simulink model "MATLAB Simulation By Lara"  (R2024a)
settings: Solver=VariableStepAuto  StartTime=0.0  StopTime=20  RelTol=1e-3
undefined symbols (not defined in the file or in its folder): Ion, Lithium
libraries: spsIdealSwitchLib x5, spsSeriesRLCBranchLib x5, instrumentseriallib x2, spsBatteryLib x1, svdutilitieslib x1, spsCurrentMeasurementLib x1, spsDCVoltageSourceLib x1, spsGroundLib x1, spsPVArrayLib x1, spsVoltageMeasurementLib x1, sps_lib x1
settings Model: Creator=LaraW  LastModifiedBy=LaraW

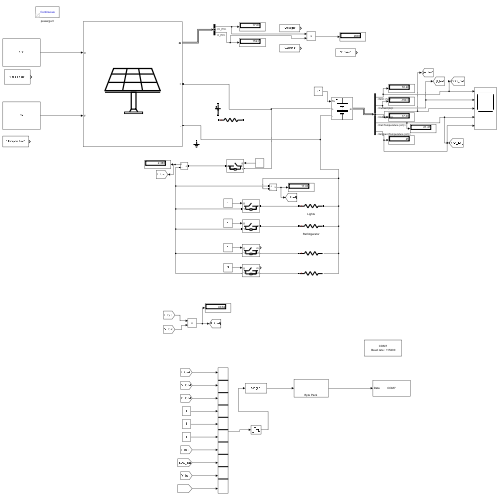
[thumbnail: Simulink's stored preview of the top-level diagram]
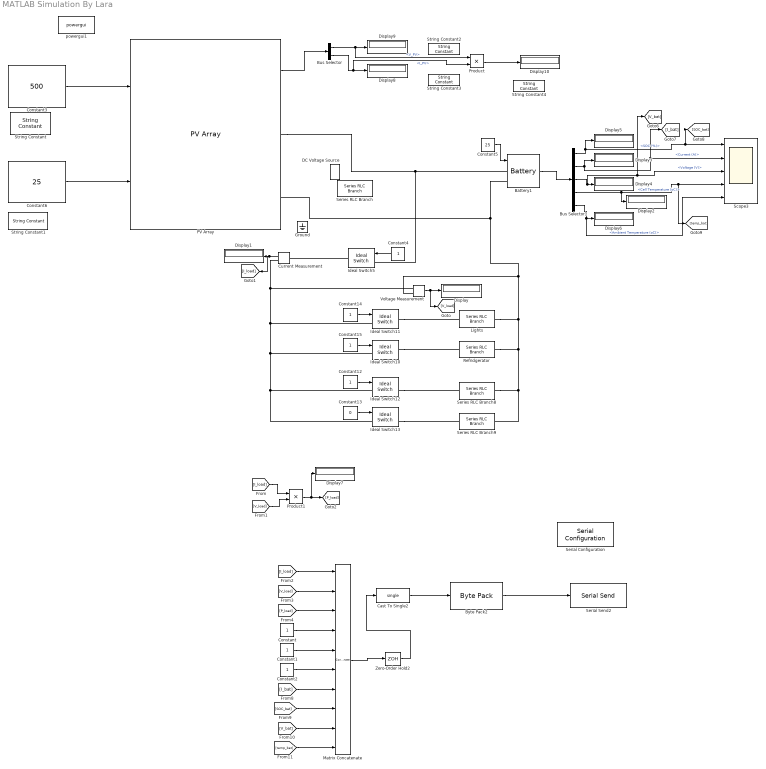
== system MATLAB Simulation By Lara ==
  Battery1 : spsBatteryLib/Battery  BatType=Lithium-Ion  ShowTempParam=on  ThermalPreset="12.8V  40Ah  (LiFeMgPO4)"  ShowAgeParam=off  NomV=12.6  NomQ=40  SOC=70  Batt_Tr=30  PresetModel=off  MaxQ=40  MinV=10.5  FullV=13.8  Dis_rate=20  R=0.015  Normal_OP=30.14  expZone="[13.1          0.5]"  current=[6.5 13 32.5]  Units=Time  Tci=20  NomT=20  T2=0  MaxQ2=36  FullV2=13  Normal_OP2=11.7  expZone2="[12.67            4]"  Rca=0.6411  ti=4880  Dp=0  Neq0=0  Tsim=1e6  Ta1=25  Qeol=5.4*0.9  Reol=0.013333*1.2  Char_age=[2.3478, 3]  Dis_age=[2.3478, 10]  N1=1500  N2=10500  N3=1000  N4=1400  Ta2=45  N5=950
  Bus Selector : BusSelector  OutputSignals=V_PV,I_PV
  Bus Selector1 : BusSelector  OutputSignals=SOC (%),Current (A),Voltage (V),Cell Temperature (oC),Ambient Temperature (oC)
  Byte Pack2 : svdutilitieslib/Byte Pack  maskPackedDataType=uint8  datatypes={'single'}  byteAlign=1  blockPlatform=arduinoert
      settings: LibrarySourceBlock=mcblib/Signal Management/Byte Pack
  Cast To Single2 : DataTypeConversion  OutDataTypeStr=single  SaturateOnIntegerOverflow=off  RndMeth=Floor
  Constant{,1..2,4,12,14..15} (7 alike) : Constant
  Constant13 : Constant  Value=0
  Constant3 : Constant  Value=500
  Constant5 : Constant  Value=25
  Constant6 : Constant  Value=25
  Current Measurement : spsCurrentMeasurementLib/Current Measurement  PhasorSimulation=off  OutputType=Complex  PSBequivalent=0
  DC Voltage Source : spsDCVoltageSourceLib/DC Voltage Source  Amplitude=12  Measurements=None
  Display{,1..10} (11 alike) : Display
  Ground : spsGroundLib/Ground  LConnTagsString=a
  Ideal Switch10 : spsIdealSwitchLib/Ideal Switch  Ron=0.001  Lon=0  IC=0  Rs=1e5  Cs=inf  Measurements=off
  Ideal Switch11 : spsIdealSwitchLib/Ideal Switch  Ron=0.001  Lon=0  IC=0  Rs=1e5  Cs=inf  Measurements=off
  Ideal Switch12 : spsIdealSwitchLib/Ideal Switch  Ron=0.001  Lon=0  IC=0  Rs=1e5  Cs=inf  Measurements=on
  Ideal Switch13 : spsIdealSwitchLib/Ideal Switch  Ron=0.001  Lon=0  IC=0  Rs=1e5  Cs=inf  Measurements=on
  Ideal Switch5 : spsIdealSwitchLib/Ideal Switch  Ron=0.001  Lon=0  IC=0  Rs=1e5  Cs=inf  Measurements=off
  Lights : spsSeriesRLCBranchLib/Series RLC Branch  LConnTagsString=__new0  RConnTagsString=__new0  BranchType=R  Resistance=16  Inductance=1e-3  SetiL0=off  InitialCurrent=0  Capacitance=1e-6  Setx0=off  InitialVoltage=0  Measurements=None
  Matrix Concatenate : Concatenate  NumInputs=10  ConcatenateDimension=2
  PV Array : spsPVArrayLib/PV Array  Npar=50  Nser=1  PlotType=array @ 1000 W/m2 & specified temperatures  S_vec="[ 1000  500  100 ]"  Temp_C_vec="[ 45 25  ]"  ModuleName=User-defined  PlotWhenSelected=off  Pm=110.25  Ncell=20  Voc=20  Isc=7.84  Vm=15  Im=7.35  beta_Voc_pc=-0.36099  alpha_Isc_pc=0.102  beta_Voc=-0.072198  alpha_Isc=0.0079968  IL=7.9228  I0=2.9127e-10  nI=1.621  Rsh=159.9332  Rs=0.36725  RobustModel=off  RobustCellTemperature=313.3991  BAL=on  Tc=1e-6  Tfilter=5e-5
  Product : Product
  Product1 : Product
  Refridgerator : spsSeriesRLCBranchLib/Series RLC Branch  LConnTagsString=__new0  RConnTagsString=__new0  BranchType=R  Resistance=12.9  Inductance=1e-3  SetiL0=off  InitialCurrent=0  Capacitance=1e-6  Setx0=off  InitialVoltage=0  Measurements=None
  Scope3 : Scope  NumInputPorts=5
  Serial Configuration : instrumentseriallib/Serial Configuration  Priority=-200000  PortSel=COM7  Port=COM7  ComPort=COM7  BaudRate=115200  DataBits=8  Parity=none  StopBits=1  ByteOrder=little-endian  FlowControl=none  Timeout=10  SimulateUsing=Interpreted execution  BlockInModel=on  aMode=1
      settings: LibrarySourceBlock=c2000lib/Host Communication/Serial Configuration
  Serial Send2 : instrumentseriallib/Serial Send  Priority=1  PortSel=COM7  Port=COM7  ComPort=COM7  Header=[]  Terminator=<none>  CustomTerminator=[]  EnableBlockingMode=on  SimulateUsing=Interpreted execution  BlockInModel=on  aMode=1
      settings: LibrarySourceBlock=c2000lib/Host Communication/Serial Send
  Series RLC Branch : spsSeriesRLCBranchLib/Series RLC Branch  LConnTagsString=__new0  RConnTagsString=__new0  BranchType=R  Resistance=3.48  Inductance=1e-3  SetiL0=off  InitialCurrent=0  Capacitance=1e-6  Setx0=off  InitialVoltage=0  Measurements=None
  Series RLC Branch8 : spsSeriesRLCBranchLib/Series RLC Branch  LConnTagsString=__new0  RConnTagsString=__new0  BranchType=R  Resistance=34000  Inductance=1e-3  SetiL0=off  InitialCurrent=0  Capacitance=1e-6  Setx0=off  InitialVoltage=0  Measurements=None
  Series RLC Branch9 : spsSeriesRLCBranchLib/Series RLC Branch  LConnTagsString=__new0  RConnTagsString=__new0  BranchType=R  Resistance=348  Inductance=1e-3  SetiL0=off  InitialCurrent=0  Capacitance=1e-6  Setx0=off  InitialVoltage=0  Measurements=None
  String Constant : StringConstant  String="\"Irradiance\""
  String Constant1 : StringConstant  String="\"Temperature\""
  String Constant2 : StringConstant  String="\"Voltage\""
  String Constant3 : StringConstant  String="\"Current\""
  String Constant4 : StringConstant  String="\"Power\""
  Voltage Measurement : spsVoltageMeasurementLib/Voltage Measurement  PhasorSimulation=off  OutputType=Complex  PSBequivalent=0
  Zero-Order Hold2 : ZeroOrderHold  SampleTime=-1
  powergui1 : sps_lib/powergui  Priority=1  SimulationMode=Continuous  SampleTime=1  frequency=60  Iterations=50  frequencyindice=0  Pbase=100e6  ErrMax=1e-4  UnitsV=kV  UnitsW=MW  buscounter=0  FunctionMessages=off  echomessages=off  EnableUseOfTLC=off  CurrentSourceSwitches=off  DisableSnubberDevices=off  DisableRonSwitches=off  DisableVfSwitches=off  DisplayEquations=off  AutomaticDiscreteSolvers=off  SolverType=Tustin/Backward Euler (TBE)  Interpol=off  ExternalGateDelay=off  methode=off  Ts=100  x0status=blocks  SPID=on  SwTol=0  HookPort=off  NonlinearTolerance=1e-4  nMaxIteration=100  ContinueOnMaxIteration=off  RestoreLinks=warning  ResistiveCurrentMeasurement=off  Frange=[0:2:500]  Ylog=off  Xlog=on  ShowGrid=off  save=off  variable=ZData  structure=0  ZoomFFT=off  StartTime=0.0  cycles=1  DisplayStyle=1  fundamental=60  FreqAxis=off  MaxFrequency=1000  frequencyindicesteady=1  RmsSteady=1  display=off
  wires:
  Bus Selector1/2 -> [I_bat], Scope3/2, Display3/1  "<Current (A)>"
  Current Measurement/1 -> [I_load], Display1/1
  Bus Selector1/4 -> Display2/1, Scope3/4, [temp_bat]  "<Cell Temperature (oC)>"
  Constant5/1 -> Battery1/1
  Constant14/1 -> Ideal Switch11/1
  Constant12/1 -> Ideal Switch12/1
  Constant15/1 -> Ideal Switch10/1
  Constant13/1 -> Ideal Switch13/1
  Constant4/1 -> Ideal Switch5/1
  Battery1/1 -> Bus Selector1/1
  Voltage Measurement/1 -> [V_load], Display/1
  Bus Selector1/1 -> Display5/1, [SOC_bat], Scope3/1  "<SOC (%)>"
  Bus Selector1/3 -> [V_bat], Scope3/3, Display4/1  "<Voltage (V)>"
  Bus Selector1/5 -> Display6/1, Scope3/5  "<Ambient Temperature (oC)>"
  Matrix Concatenate/1 -> Zero-Order Hold2/1
  Cast To Single2/1 -> Byte Pack2/1
  Byte Pack2/1 -> Serial Send2/1
  Zero-Order Hold2/1 -> Cast To Single2/1
  [temp_bat] -> Matrix Concatenate/10
  Constant1/1 -> Matrix Concatenate/5
  [V_load] -> Product1/2
  [I_bat] -> Matrix Concatenate/7
  [V_load] -> Matrix Concatenate/2
  Product1/1 -> Display7/1, [P_load]
  [SOC_bat] -> Matrix Concatenate/8
  [I_load] -> Matrix Concatenate/1
  Constant/1 -> Matrix Concatenate/4
  [P_load] -> Matrix Concatenate/3
  [I_load] -> Product1/1
  [V_bat] -> Matrix Concatenate/9
  Constant2/1 -> Matrix Concatenate/6
  Product/1 -> Display10/1
  PV Array/1 -> Bus Selector/1
  Bus Selector/2 -> Display8/1, Product/2  "<I_PV>"
  Constant6/1 -> PV Array/2
  Constant3/1 -> PV Array/1
  Bus Selector/1 -> Display9/1, Product/1  "<V_PV>"
  connections:
  Voltage Measurement/LConn1 -- Ideal Switch13/LConn1 -- Ideal Switch12/LConn1 -- Ideal Switch10/LConn1 -- Ideal Switch11/LConn1 -- Current Measurement/RConn1
  Ideal Switch13/RConn1 -- Series RLC Branch9/LConn1
  Ideal Switch12/RConn1 -- Series RLC Branch8/LConn1
  Ideal Switch10/RConn1 -- Refridgerator/LConn1
  Ideal Switch11/RConn1 -- Lights/LConn1
  Ideal Switch5/RConn1 -- Current Measurement/LConn1
  Voltage Measurement/LConn2 -- Lights/RConn1 -- Refridgerator/RConn1 -- Series RLC Branch8/RConn1 -- Series RLC Branch9/RConn1 -- PV Array/RConn2 -- Battery1/LConn2
  PV Array/RConn1 -- Battery1/LConn1 -- Ideal Switch5/LConn1
